simulink model "VelocityEstimator_Example"  (Simulink 8.2)
settings: Solver=FixedStepDiscrete  StartTime=0.0  StopTime=8  FixedStep=Ts  RelTol=1e-3
PreLoadFcn:
  | Ts = 0.001
undefined symbols (not defined in the file or in its folder): DiscIntNeverNeededParam
libraries: simulink x2
settings Model: Creator=Luke  LastModifiedBy=LukePH
settings DataIOCC: SignalLoggingSaveFormat=Dataset
settings DebuggingCC: FcnCallInpInsideContextMsg=EnableAllAsError
settings GRTTargetCC: CombineOutputUpdateFcns=on  GRTInterface=off

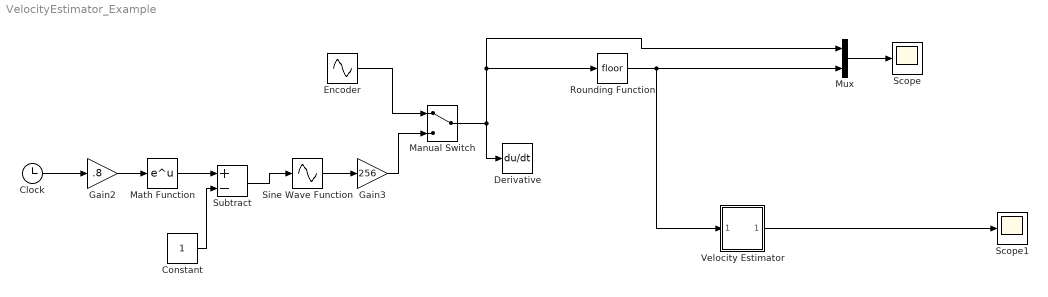
== system VelocityEstimator_Example ==
  Clock : Clock
  Constant : Constant
  Derivative : Derivative
  Encoder : Sin  Amplitude=1024  Bias=0.001  Frequency=pi/2  SampleTime=0
  Gain2 : Gain  Gain=.8
  Gain3 : Gain  Gain=256
  Manual Switch : ManualSwitch
  Math Function : Math  SaturateOnIntegerOverflow=on
  Mux : Mux  Inputs=2
  Rounding Function : Rounding
  Scope : Scope
  Scope1 : Scope
  Sine Wave Function : Sin  TimeSource=Use external signal  SampleTime=0
  Subtract : Sum  Inputs=+-
  Velocity Estimator : Subsystem  mask{SampleTime=Ts}
      mask prompts: SampleTime "Sample time (-1 for inherited):"
      mask help:
      | This Block takes in encoder values at a rate of 1 sample per Ts seconds and
      | produces an estimate of the velocity at the given time.
      mask TypeOptions SampleTime: Velocity /SystemSampleTime | Weight Calc/SystemSampleTime | Weighted Average/SystemSampleTime | Velocity /Time Constant/Value | Discrete-Time Integrator/SampleTime | Dead Zone/SampleTime | Weight Calc/9000 rad//sec^2 Cut-off/SampleTime | Weight Calc/Discrete Low Pass1/SampleTime | Weight Calc/Discrete Transfer Fcn/SampleTime | Weight Calc/Discrete Transfer Fcn1/SampleTime | Discrete Low Pass2/SampleTime | Velocity /My Difference/Delay/SampleTime | Velocity /My Difference/Sum/SampleTime
      mask Display:
      | port_label('output', 1, '')
      | port_label('input', 1, '')
  wires:
  Mux/1 -> Scope/1
  Manual Switch/1 -> Derivative/1, Rounding Function/1, Mux/1
  Encoder/1 -> Manual Switch/1
  Clock/1 -> Gain2/1
  Gain2/1 -> Math Function/1
  Gain3/1 -> Manual Switch/2
  Sine Wave Function/1 -> Gain3/1
  Math Function/1 -> Subtract/1
  Subtract/1 -> Sine Wave Function/1
  Constant/1 -> Subtract/2
  Rounding Function/1 -> Velocity Estimator/1(In1), Mux/2
  Velocity Estimator/1(Out1) -> Scope1/1

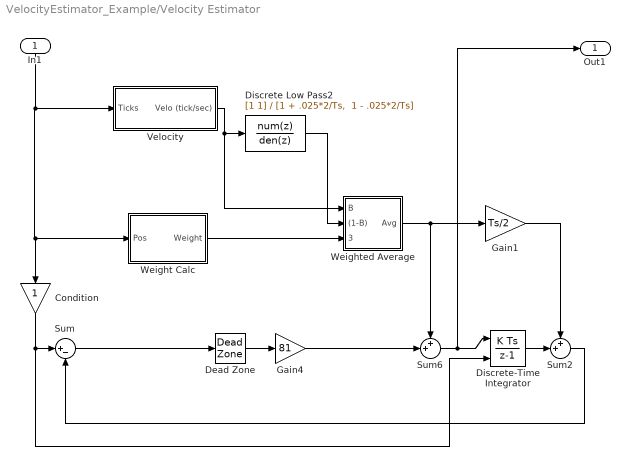
== system VelocityEstimator_Example/Velocity Estimator ==
  In1 : Inport
  Condition : Gain  OutMin=0  OutMax=10^9  OutDataTypeStr=double
  Dead Zone : DeadZone  LowerValue=-1  UpperValue=1  SampleTime=SampleTime  SaturateOnIntegerOverflow=on
  Discrete Low Pass2 : DiscreteTransferFcn  Numerator=[1 1]  Denominator="[1 + .025*2/Ts,  1 - .025*2/Ts]"  SampleTime=SampleTime
  Discrete-Time Integrator : DiscreteIntegrator  InitialConditionSource=external  SampleTime=SampleTime  ICPrevOutput=DiscIntNeverNeededParam  ICPrevScaledInput=DiscIntNeverNeededParam
  Gain1 : Gain  Gain=Ts/2
  Gain4 : Gain  Gain=81
  Sum : Sum  Inputs=|+-
  Sum2 : Sum  Inputs=++|
  Sum6 : Sum  Inputs=++|
  "Velocity " : Subsystem  SystemSampleTime=SampleTime
  Weight Calc : Subsystem  SystemSampleTime=SampleTime
  Weighted Average : Subsystem  SystemSampleTime=SampleTime
  Out1 : Outport
  wires:
  Weight Calc/1(Weight) -> Weighted Average/3(Weight)
  Gain1/1 -> Sum2/1
  Discrete-Time Integrator/1 -> Sum2/2
  Sum2/1 -> Sum/2
  Discrete Low Pass2/1 -> Weighted Average/2((1-B))
  Sum6/1 -> Out1/1, Discrete-Time Integrator/1
  Dead Zone/1 -> Gain4/1
  Weighted Average/1(Avg) -> Sum6/1, Gain1/1
  Gain4/1 -> Sum6/2
  Sum/1 -> Dead Zone/1
  "Velocity "/1(Velo (tick/sec)) -> Weighted Average/1("B "), Discrete Low Pass2/1
  In1/1 -> Condition/1, Weight Calc/1(Pos), "Velocity "/1(Ticks)
  Condition/1 -> Discrete-Time Integrator/2, Sum/1

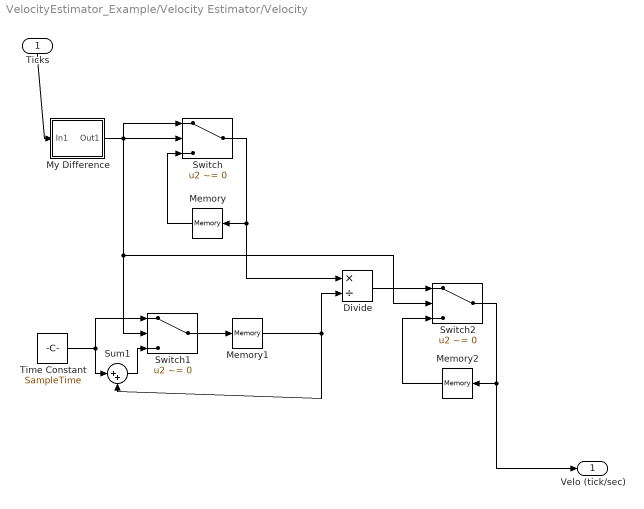
== system VelocityEstimator_Example/Velocity Estimator/Velocity  ==
  Ticks : Inport  SampleTime=Ts
  Divide : Product  Inputs=*/
  Memory : Memory
  Memory1 : Memory  X0=Ts
  Memory2 : Memory
  My Difference : Subsystem
  Sum1 : Sum  Inputs=|++
  Switch : Switch  Criteria=u2 ~= 0
  Switch1 : Switch  Criteria=u2 ~= 0
  Switch2 : Switch  Criteria=u2 ~= 0
  Time Constant : Constant  Value=SampleTime
  Velo (tick/sec) : Outport  SampleTime=Ts
  wires:
  Ticks/1 -> My Difference/1(In1)
  My Difference/1(Out1) -> Switch/1, Switch1/2, Switch2/2, Switch/2
  Switch/1 -> Divide/1, Memory/1
  Memory/1 -> Switch/3
  Switch1/1 -> Memory1/1
  Time Constant/1 -> Switch1/1, Sum1/1
  Sum1/1 -> Switch1/3
  Memory1/1 -> Sum1/2, Divide/2
  Divide/1 -> Switch2/1
  Memory2/1 -> Switch2/3
  Switch2/1 -> Velo (tick/sec)/1, Memory2/1

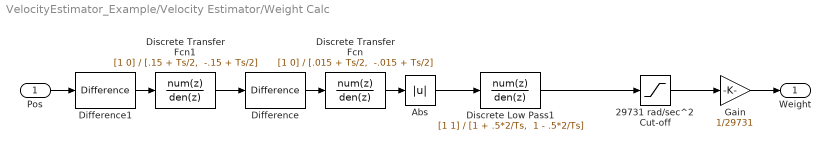
== system VelocityEstimator_Example/Velocity Estimator/Weight Calc ==
  Pos : Inport
  29731 rad/sec^2 Cut-off : Saturate  UpperLimit=29731  LowerLimit=0  SampleTime=SampleTime
  Abs : Abs  OutMin=0  OutMax=10^9  OutDataTypeStr=fixdt(1,16)
  Difference : simulink/Discrete/Difference  ICPrevInput=0.0  InputProcessing=Inherited  OutMin=[]  OutMax=[]  OutDataType=fixdt(1, 16)  OutScaling=2^-10  DoSatur=off
  Difference1 : simulink/Discrete/Difference  ICPrevInput=0.0  InputProcessing=Inherited  OutMin=[]  OutMax=[]  OutDataType=fixdt(1, 16)  OutScaling=2^-10  DoSatur=off
  Discrete Low Pass1 : DiscreteTransferFcn  Numerator=[1 1]  Denominator="[1 + .5*2/Ts,  1 - .5*2/Ts]"  SampleTime=SampleTime
  Discrete Transfer Fcn : DiscreteTransferFcn  Numerator=[1 0]  Denominator="[.015 + Ts/2,  -.015 + Ts/2]"  SampleTime=SampleTime
  Discrete Transfer Fcn1 : DiscreteTransferFcn  Numerator=[1 0]  Denominator="[.15 + Ts/2,  -.15 + Ts/2]"  SampleTime=SampleTime
  Gain : Gain  Gain=1/29731
  Weight : Outport  SampleTime=Ts
  wires:
  Gain/1 -> Weight/1
  29731 rad/sec^2 Cut-off/1 -> Gain/1
  Difference1/1 -> Discrete Transfer Fcn1/1
  Difference/1 -> Discrete Transfer Fcn/1
  Discrete Transfer Fcn1/1 -> Difference/1
  Pos/1 -> Difference1/1
  Discrete Transfer Fcn/1 -> Abs/1
  Abs/1 -> Discrete Low Pass1/1
  Discrete Low Pass1/1 -> 29731 rad/sec^2 Cut-off/1

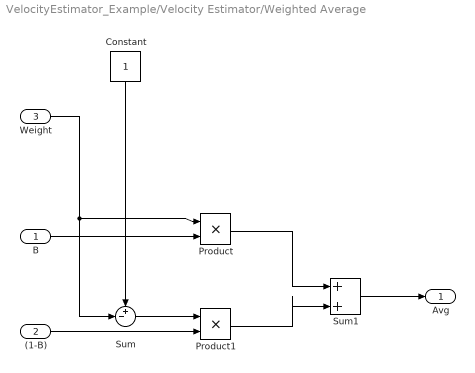
== system VelocityEstimator_Example/Velocity Estimator/Weighted Average ==
  "B " : Inport
  (1-B) : Inport  Port=2
  Weight : Inport  Port=3
  Constant : Constant
  Product : Product  RndMeth=Zero
  Product1 : Product  RndMeth=Zero
  Sum : Sum  Inputs=+-|
  Sum1 : Sum  Inputs=++|
  Avg : Outport
  wires:
  "B "/1 -> Product/2
  Weight/1 -> Product/1, Sum/2
  (1-B)/1 -> Product1/2
  Constant/1 -> Sum/1
  Sum/1 -> Product1/1
  Product1/1 -> Sum1/2
  Product/1 -> Sum1/1
  Sum1/1 -> Avg/1

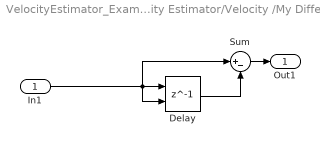
== system VelocityEstimator_Example/Velocity Estimator/Velocity /My Difference ==
  In1 : Inport
  Delay : Delay  DelayLength=1  InitialConditionSource=Input port  SampleTime=Ts
      settings: InputPortMap=u0,p4
  Sum : Sum  Inputs=|+-  SampleTime=Ts
  Out1 : Outport
  wires:
  In1/1 -> Delay/2, Sum/1, Delay/1
  Sum/1 -> Out1/1
  Delay/1 -> Sum/2
